simulink model "Duplicat_Test"  (R2025b)
settings: Solver=FixedStepAuto  StartTime=0.0  StopTime=inf  RelTol=1e-3
settings Model: SimulationMode=external  Creator=kueh_js  LastModifiedBy=kueh_js
settings OptimizationCC: OptimizeBlockIOStorage=off  EnhancedBackFolding=on  PassReuseOutputArgsThreshold=0.0  ZeroExternalMemoryAtStartup=off  ZeroInternalMemoryAtStartup=off  OptimizeBlockOrder=speed  DifferentSizesBufferReuse=on
settings DebuggingCC: ParameterTunabilityLossMsg=error
settings HardwareCC: ProdBitPerLong=64.0  ProdHWDeviceType=Intel->x86-64 (Linux 64)
settings SFSimCC: MATLABDynamicMemAlloc=off  SimTargetLang=C++  SimDLTargetLibrary=mkl-dnn
settings RTWCC: GenCodeOnly=on  Toolchain=GNU gcc/g++ | gmake (64-bit Linux)  TargetLang=C++
settings CodeAppCC: ForceParamTrailComments=on  OperatorAnnotations=on  MATLABSourceComments=on
settings GRTTargetCC: TargetLangStandard=C++20 (ISO)  MatFileLogging=off  CodeInterfacePackaging=C++ class

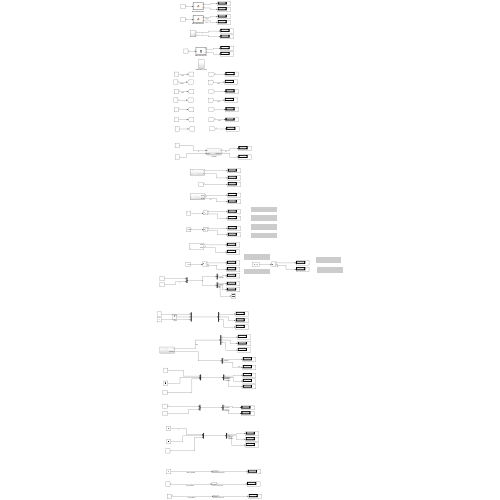
[thumbnail: Simulink's stored preview of the top-level diagram]
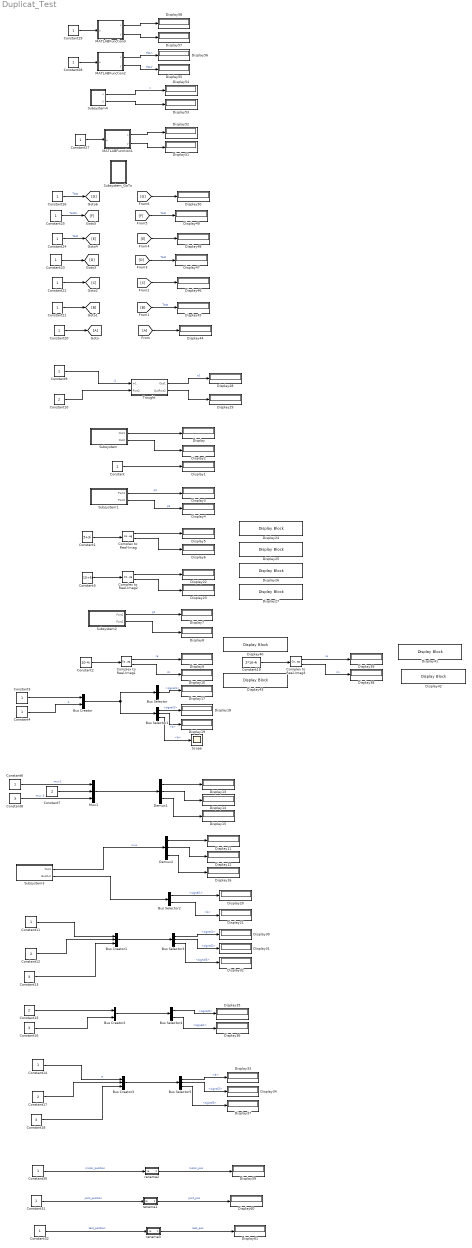
== system Duplicat_Test ==
  Bus Creator : BusCreator  Inputs=2
  Bus Creator1 : BusCreator  Inputs=3
  Bus Creator2 : BusCreator  Inputs=2
  Bus Creator3 : BusCreator  Inputs=3
  Bus Selector : BusSelector  OutputSignals=signal1
  Bus Selector1 : BusSelector  OutputSignals=signal1,b,b
  Bus Selector2 : BusSelector  OutputSignals=signal1,b
  Bus Selector3 : BusSelector  OutputSignals=signal1,signal2,signal3
  Bus Selector4 : BusSelector  OutputSignals=signal2,signal1
  Bus Selector5 : BusSelector  OutputSignals=a,signal2,signal3
  Complex to Real-Imag{,1..3} (4 alike) : ComplexToRealImag
  Constant{,3..4,6,9,11,14,20..32} (20 alike) : Constant
  Constant1 : Constant  Value=5+3i
  Constant{7,10,12,15,17} (5 alike) : Constant  Value=2
  Constant{8,13,16,18} (4 alike) : Constant  Value=3
  Constant19 : Constant  Value=2*10-4i
  Constant2 : Constant  Value=10-4i
  Constant5 : Constant  Value=10+6i
  Demux1 : Demux  Outputs=3
  Demux2 : Demux  Outputs=3
  Display{,1..23,28..39,44..61} (54 alike) : Display
  Display{24..27,40..43} (8 alike) : DisplayBlock  LabelPosition=Hide  Transparency=1  GridColor=[0.502, 0.502, 0.502]
  From : From
  Goto : Goto
  MATLABFunction1 : MATLAB Function  TreatAsAtomicUnit=on
  MATLABFunction2 : MATLAB Function  TreatAsAtomicUnit=on
  MATLABFunction3 : MATLAB Function  TreatAsAtomicUnit=on
  Mux1 : Mux  Inputs=3
  Scope : Scope
  Subsystem : Subsystem
  Subsystem1 : Subsystem
  Subsystem2 : Subsystem  mask{dof=5}
  Subsystem3 : Subsystem
  Subsystem4 : Subsystem
  Subsystem_GoTo : Subsystem
  Trought : Subsystem
  rename1 : Subsystem
  rename2 : Subsystem
  rename3 : Subsystem
  wires:
  Complex to Real-Imag/1 -> Display5/1
  Constant1/1 -> Complex to Real-Imag/1
  Subsystem1/2(Port2) -> Display4/1  "p2"
  Subsystem2/2(Port2) -> Display8/1
  Subsystem1/1(Port1) -> Display3/1  "p1"
  Constant/1 -> Display1/1
  Complex to Real-Imag/2 -> Display6/1
  Subsystem/2(Out2) -> Display2/1
  Subsystem2/1(Port1) -> Display7/1  "p1"
  Subsystem/1(Out1) -> Display/1
  Complex to Real-Imag1/1 -> Display9/1  "re"
  Complex to Real-Imag1/2 -> Display10/1  "im"
  Constant2/1 -> Complex to Real-Imag1/1
  Constant7/1 -> Mux1/2
  Constant8/1 -> Mux1/3  "mux 3"
  Demux1/1 -> Display13/1
  Constant6/1 -> Mux1/1  "mux1"
  Demux1/2 -> Display14/1
  Mux1/1 -> Demux1/1
  Demux1/3 -> Display15/1
  Demux2/1 -> Display11/1
  Demux2/2 -> Display12/1
  Demux2/3 -> Display16/1
  Subsystem3/1(Out1) -> Demux2/1  "mux"
  Bus Creator/1 -> Bus Selector1/1, Bus Selector/1
  Constant3/1 -> Bus Creator/1
  Constant4/1 -> Bus Creator/2  "b"
  Bus Selector/1 -> Display17/1  "<signal1>"
  Bus Selector1/1 -> Display18/1  "<signal1>"
  Bus Selector1/2 -> Display19/1  "<b>"
  Bus Selector1/3 -> Scope/1  "<b>"
  Subsystem3/2(BusOut) -> Bus Selector2/1
  Bus Selector2/1 -> Display20/1  "<signal1>"
  Bus Selector2/2 -> Display21/1  "<b>"
  Complex to Real-Imag2/1 -> Display22/1
  Constant5/1 -> Complex to Real-Imag2/1
  Complex to Real-Imag2/2 -> Display23/1
  Constant9/1 -> Trought/1(In1)  "i1"
  Constant10/1 -> Trought/2(Port2)
  Trought/1(Out1) -> Display28/1  "o1"
  Trought/2(OutPort2) -> Display29/1
  Bus Creator1/1 -> Bus Selector3/1
  Constant11/1 -> Bus Creator1/1
  Constant12/1 -> Bus Creator1/2
  Constant13/1 -> Bus Creator1/3
  Bus Selector3/1 -> Display30/1  "<signal1>"
  Bus Selector3/2 -> Display31/1  "<signal2>"
  Bus Selector3/3 -> Display32/1  "<signal3>"
  Bus Selector4/1 -> Display35/1  "<signal2>"
  Constant16/1 -> Bus Creator2/2
  Bus Creator2/1 -> Bus Selector4/1
  Constant15/1 -> Bus Creator2/1
  Bus Selector4/2 -> Display36/1  "<signal1>"
  Bus Selector5/2 -> Display34/1  "<signal2>"
  Constant18/1 -> Bus Creator3/3
  Bus Selector5/1 -> Display33/1  "<a>"
  Bus Creator3/1 -> Bus Selector5/1
  Constant17/1 -> Bus Creator3/2
  Bus Selector5/3 -> Display37/1  "<signal3>"
  Constant14/1 -> Bus Creator3/1  "a"
  Constant19/1 -> Complex to Real-Imag3/1
  Complex to Real-Imag3/1 -> Display39/1  "re"
  Complex to Real-Imag3/2 -> Display38/1  "im"
  From/1 -> Display44/1
  Constant20/1 -> Goto/1
  [B] -> Display45/1  "Test"
  Constant21/1 -> [B]
  Constant23/1 -> [D]
  [C] -> Display46/1
  [D] -> Display47/1  "Test"
  Constant22/1 -> [C]
  Constant24/1 -> [E]  "Test"
  Constant25/1 -> [F]  "TestIn"
  [E] -> Display48/1
  [F] -> Display49/1  "Test"
  Constant26/1 -> [G]  "Test"
  [G] -> Display50/1
  Constant27/1 -> MATLABFunction1/1(u)
  MATLABFunction1/2(y) -> Display51/1
  MATLABFunction1/1(x) -> Display52/1
  Subsystem4/1(x) -> Display54/1  "x"
  Subsystem4/2(y) -> Display53/1
  MATLABFunction2/1(x) -> Display56/1  "sig_x"
  MATLABFunction2/2(y) -> Display55/1  "sig_y"
  Constant28/1 -> MATLABFunction2/1(u)
  MATLABFunction3/1(x) -> Display58/1
  MATLABFunction3/2(y) -> Display57/1
  Constant29/1 -> MATLABFunction3/1(u)
  Constant30/1 -> rename2/1(re)  "motor_position"
  rename2/1(name) -> Display59/1  "motor_pos"
  rename1/1(name) -> Display60/1  "joint_pos"
  Constant31/1 -> rename1/1(re)  "joint_position"
  Constant32/1 -> rename3/1(re)  "test_position"
  rename3/1(name) -> Display61/1  "test_pos"

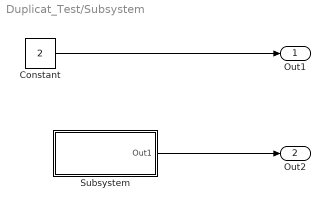
== system Duplicat_Test/Subsystem ==
  Constant : Constant  Value=2
  Subsystem : Subsystem
  Out1 : Outport
  Out2 : Outport  Port=2
  wires:
  Constant/1 -> Out1/1
  Subsystem/1(Out1) -> Out2/1

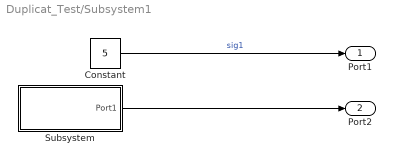
== system Duplicat_Test/Subsystem1 ==
  Constant : Constant  Value=5
  Subsystem : Subsystem
  Port1 : Outport
  Port2 : Outport  Port=2
  wires:
  Constant/1 -> Port1/1  "sig1"
  Subsystem/1(Port1) -> Port2/1

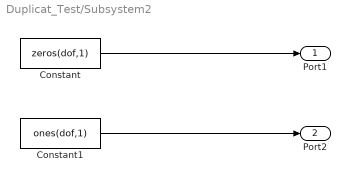
== system Duplicat_Test/Subsystem2 ==
  Constant : Constant  Value=zeros(dof,1)
  Constant1 : Constant  Value=ones(dof,1)
  Port1 : Outport
  Port2 : Outport  Port=2
  wires:
  Constant/1 -> Port1/1
  Constant1/1 -> Port2/1

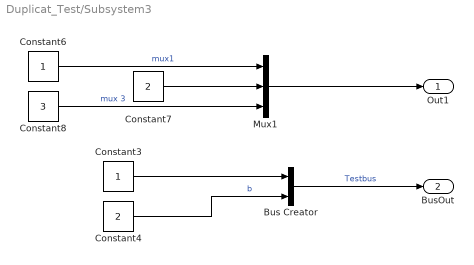
== system Duplicat_Test/Subsystem3 ==
  Bus Creator : BusCreator  Inputs=2
  Constant3 : Constant
  Constant4 : Constant  Value=2
  Constant6 : Constant
  Constant7 : Constant  Value=2
  Constant8 : Constant  Value=3
  Mux1 : Mux  Inputs=3
  Out1 : Outport
  BusOut : Outport  Port=2
  wires:
  Mux1/1 -> Out1/1
  Constant6/1 -> Mux1/1  "mux1"
  Constant8/1 -> Mux1/3  "mux 3"
  Constant7/1 -> Mux1/2
  Constant3/1 -> Bus Creator/1
  Constant4/1 -> Bus Creator/2  "b"
  Bus Creator/1 -> BusOut/1  "Testbus"

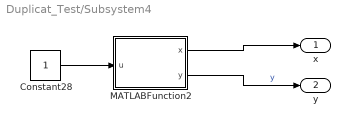
== system Duplicat_Test/Subsystem4 ==
  Constant28 : Constant
  MATLABFunction2 : MATLAB Function  TreatAsAtomicUnit=on
  x : Outport
  y : Outport  Port=2
  wires:
  Constant28/1 -> MATLABFunction2/1(u)
  MATLABFunction2/2(y) -> y/1  "y"
  MATLABFunction2/1(x) -> x/1

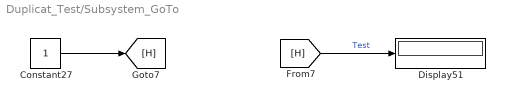
== system Duplicat_Test/Subsystem_GoTo ==
  Constant27 : Constant
  Display51 : Display
  wires:
  Constant27/1 -> [H]
  [H] -> Display51/1  "Test"

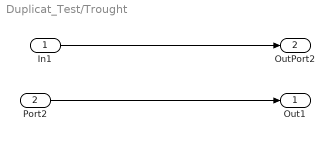
== system Duplicat_Test/Trought ==
  In1 : Inport
  Port2 : Inport  Port=2
  Out1 : Outport
  OutPort2 : Outport  Port=2
  wires:
  In1/1 -> OutPort2/1
  Port2/1 -> Out1/1

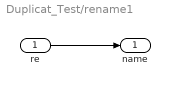
== system Duplicat_Test/rename1 ==
  re : Inport
  name : Outport  VectorParamsAs1DForOutWhenUnconnected=off
  wires:
  re/1 -> name/1

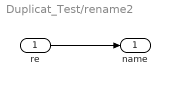
== system Duplicat_Test/rename2 ==
  re : Inport
  name : Outport  VectorParamsAs1DForOutWhenUnconnected=off
  wires:
  re/1 -> name/1

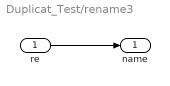
== system Duplicat_Test/rename3 ==
  re : Inport
  name : Outport  VectorParamsAs1DForOutWhenUnconnected=off
  wires:
  re/1 -> name/1

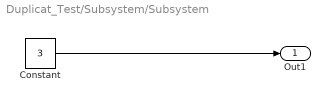
== system Duplicat_Test/Subsystem/Subsystem ==
  Constant : Constant  Value=3
  Out1 : Outport
  wires:
  Constant/1 -> Out1/1

== system Duplicat_Test/Subsystem1/Subsystem ==
  Constant : Constant  Value=10
  Port1 : Outport
  wires:
  Constant/1 -> Port1/1

== matlab function Duplicat_Test/MATLABFunction1 ==
  data: x output; u input; y output; c parameter
function [x,y] = fcn(u,c)

y = 2*u + c;
x = c*u;

== matlab function Duplicat_Test/MATLABFunction2 ==
  data: x output; u input; y output; c parameter
function [x,y] = fcn(u,c)

y = 2*u + c;
x = c*u;

== matlab function Duplicat_Test/MATLABFunction3 ==
  data: x output; u input; y output
function [x,y] = fcn(u)

y = 2*u + 5;
x = 3*u;

== matlab function Duplicat_Test/Subsystem4/MATLABFunction2 ==
  data: x output; u input; y output; c parameter
function [x,y] = fcn(u,c)

y = 2*u + c;
x = c*u;
